simulink model "sampleModel265"  (R2021b)
settings: Solver=VariableStepAuto  StartTime=0.0  StopTime=10.0  RelTol=1e-3
undefined symbols (not defined in the file or in its folder): DiscIntNeverNeededParam, Newton, Raphson
libraries: simulink x9, slpidlib x1
settings Model: Creator=user  LastModifiedBy=user

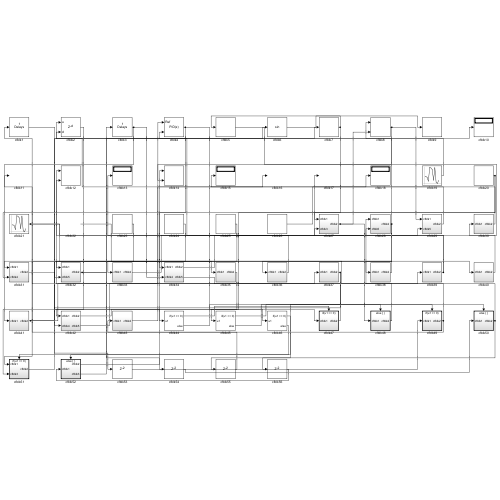
[thumbnail: Simulink's stored preview of the top-level diagram]
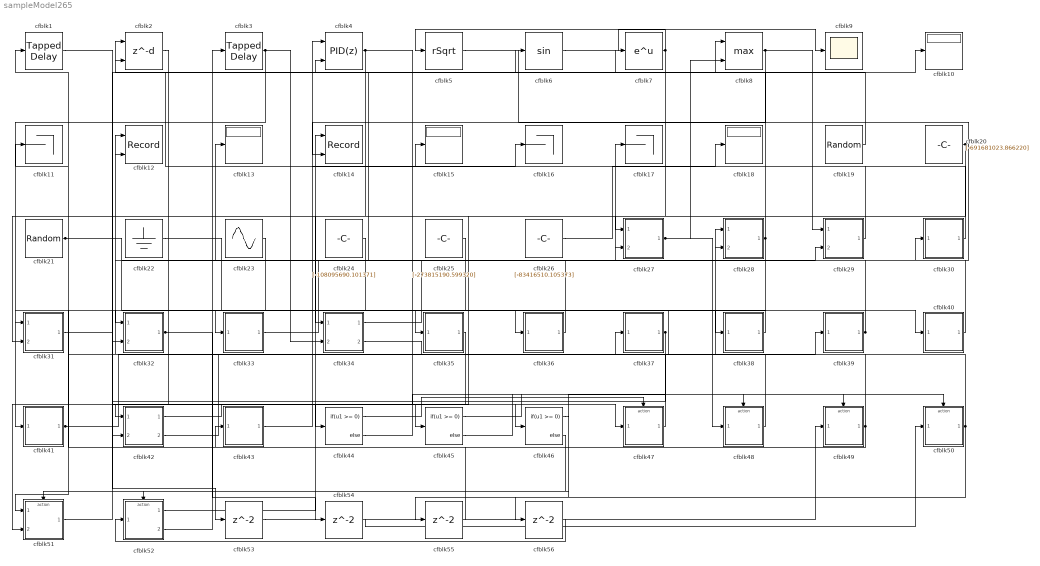
== system sampleModel265 ==
  cfblk1 : simulink/Discrete/Tapped Delay  vinit=0.0  samptime=-1  NumDelays=1  DelayOrder=Oldest  includeCurrent=off
  cfblk{10,13,15,18} (4 alike) : Display
  cfblk11 : Terminator
  cfblk12 : Record  FileSettingsInternal="{\"entries\":[{\"content\":{\"excelSettings\":{\"content\":{},\"type\":\"Streamout.ExcelSettings\"}},\"type\":\"Streamout.FileSettingStorage\",\"uuid\":\"94a5c3c0-ca64-4e36-ac7f-d04636a5f23d\"}],\"packageUris\":[\"http://schema.mathworks.com/mf0/streamout_blocks/R2020a\"],\"version\":\"1.0\"}"  Layout=[1 1]  SignalsInternal="{\"entries\":[{\"content\":{\"signals\":[{\"content\":{\"blockPath\":[\"sampleModel265/cfblk12\"],\"channel\":[],\"dimensions\":[1],\"domain\":\"sampleModel265/cfblk12\",\"lineColor\":\"#a2142f\",\"plots\":[1],\"port\":1,\"sid\":[\"\"],\"signalID\":11021,\"signalName\":\"cfblk47\"},\"type\":\"RecordBlkView.Signal\",\"uuid\":\"85f619e6-c166-47fc-b281-92095b2e0ded\"},{\"content\":{\"blockPath\":[\"sampleModel265/cfblk12\"],\"channel\":[],\"dimensions\":[1],\"domain\":\"sampleModel265/cfblk12\",\"lineColor\":\"#139fff\",\"plots\":[1],\"port\":2,\"sid\":[\"\"],\"signalID\":11025,\"signalName\":\"cfblk40\"},\"type\":\"RecordBlkView.Signal\",\"uuid\":\"cdf1bb3a-11ff-4296-b8df-4a9dbd689937\"}]},\"type\":\"RecordBlkView.InputSignals\",\"uuid\":\"aee0d6e9-f41f-4389-b4de-0f8d12f61657\"}],\"packageUris\":[\"http://schema.mathworks.com/mf0/streamout_blocks/R2020a\"],\"version\":\"1.0\"}"  VisualizationBindings="{\"xyplotplugin\":{\"info\":[{\"series\":[{\"bindingParametersList\":[{\"parameter\":\"X-Axis\",\"signalID\":11021,\"signalName\":\"cfblk47\"},{\"parameter\":\"Y-Axis\",\"signalID\":11025,\"signalName\":\"cfblk40\"}],\"seriesID\":38759}],\"subplotID\":1}]}}"  CompatibilityTag=XY
  cfblk14 : Record  FileSettingsInternal="{\"entries\":[{\"content\":{\"excelSettings\":{\"content\":{},\"type\":\"Streamout.ExcelSettings\"}},\"type\":\"Streamout.FileSettingStorage\",\"uuid\":\"8704c8db-9a0e-4fec-bce2-c10549bc8203\"}],\"packageUris\":[\"http://schema.mathworks.com/mf0/streamout_blocks/R2020a\"],\"version\":\"1.0\"}"  Layout=[1 1]  SignalsInternal="{\"entries\":[{\"content\":{\"signals\":[{\"content\":{\"blockPath\":[\"sampleModel265/cfblk14\"],\"channel\":[],\"dimensions\":[1],\"domain\":\"sampleModel265/cfblk14\",\"lineColor\":\"#a2142f\",\"plots\":[1],\"port\":1,\"sid\":[\"\"],\"signalID\":11029,\"signalName\":\"cfblk52:1\"},\"type\":\"RecordBlkView.Signal\",\"uuid\":\"9f14bc3c-b124-479f-9d7d-5ec5307796c1\"},{\"content\":{\"blockPath\":[\"sampleModel265/cfblk14\"],\"channel\":[],\"dimensions\":[1],\"domain\":\"sampleModel265/cfblk14\",\"lineColor\":\"#139fff\",\"plots\":[1],\"port\":2,\"sid\":[\"\"],\"signalID\":11033,\"signalName\":\"cfblk8\"},\"type\":\"RecordBlkView.Signal\",\"uuid\":\"a3cd0ba9-c32c-4abe-85ac-9eba25fc91aa\"}]},\"type\":\"RecordBlkView.InputSignals\",\"uuid\":\"c0d32c16-2111-47bb-aa87-fac3f9eeb510\"}],\"packageUris\":[\"http://schema.mathworks.com/mf0/streamout_blocks/R2020a\"],\"version\":\"1.0\"}"  VisualizationBindings="{\"xyplotplugin\":{\"info\":[{\"series\":[{\"bindingParametersList\":[{\"parameter\":\"X-Axis\",\"signalID\":11029,\"signalName\":\"cfblk52:1\"},{\"parameter\":\"Y-Axis\",\"signalID\":11033,\"signalName\":\"cfblk8\"}],\"seriesID\":46910}],\"subplotID\":1}]}}"  CompatibilityTag=XY
  cfblk16 : Terminator
  cfblk17 : Terminator
  cfblk19 : RandomNumber  Mean=[-17684.841578]  Variance=[64763.330717]  Seed=[934609408.000000]  SampleTime=0.1
  cfblk2 : Delay  DelayLengthSource=Input port  SampleTime=1
      settings: InputPortMap=u0,p1
  cfblk20 : Constant  Value=[-691681023.866220]  SampleTime=1
  cfblk21 : RandomNumber  Mean=[42362.461850]  Variance=[21600.172597]  Seed=[389411026.000000]  SampleTime=0.1
  cfblk22 : Ground
  cfblk23 : Sin  Amplitude=[904038054.961735]  Bias=[-430535881.463050]  SampleTime=0
  cfblk24 : Constant  Value=[-108095690.101371]  SampleTime=1
  cfblk25 : Constant  Value=[-273815190.599320]  SampleTime=1
  cfblk26 : Constant  Value=[-83416510.105373]  SampleTime=1
  cfblk27 : Subsystem
  cfblk28 : Subsystem
  cfblk29 : Subsystem
  cfblk3 : simulink/Discrete/Tapped Delay  vinit=0.0  samptime=-1  NumDelays=1  DelayOrder=Oldest  includeCurrent=off
  cfblk30 : Subsystem
  cfblk31 : Subsystem
  cfblk32 : Subsystem
  cfblk33 : Subsystem
  cfblk34 : Subsystem
  cfblk35 : Subsystem
  cfblk36 : Subsystem
  cfblk37 : Subsystem
  cfblk38 : Subsystem
  cfblk39 : Subsystem
  cfblk4 : slpidlib/PID Controller (2DOF)  Controller=PID  Form=Parallel  TimeDomain=Discrete-time  UseExternalTs=off  SampleTime=1  IntegratorMethod=Forward Euler  FilterMethod=Forward Euler  ControllerParametersSource=internal  P=1  I=1  D=0  UseFilter=on  N=100  b=1  c=1  TunerSelectOption=Transfer Function Based (PID Tuner App)  InitialConditionSource=internal  InitialConditionForIntegrator=0  InitialConditionForFilter=0  DifferentiatorICPrevScaledInput=0  ExternalReset=none  TrackingMode=off  Kt=1  LimitOutput=off  SatLimitsSource=internal  UpperSaturationLimit=inf  LowerSaturationLimit=-inf  LinearizeAsGain=off  AntiWindupMode=none  Kb=1  POutMin=[]  POutMax=[]  IOutMin=[]  IOutMax=[]  DOutMin=[]  DOutMax=[]  NOutMin=[]  NOutMax=[]  bOutMin=[]  bOutMax=[]  cOutMin=[]  cOutMax=[]  SumOutMin=[]  SumOutMax=[]  SaturationOutMin=[]  SaturationOutMax=[]  PParamMin=[]  PParamMax=[]  IParamMin=[]  IParamMax=[]  DParamMin=[]  DParamMax=[]  NParamMin=[]  NParamMax=[]  bParamMin=[]  bParamMax=[]  cParamMin=[]  cParamMax=[]  KbParamMin=[]  KbParamMax=[]  KtParamMin=[]  KtParamMax=[]  KbOutMin=[]  KbOutMax=[]  KtOutMin=[]  KtOutMax=[]  IntegratorOutMin=[]  IntegratorOutMax=[]  FilterOutMin=[]  FilterOutMax=[]  SumI1OutMin=[]  SumI1OutMax=[]  SumI2OutMin=[]  SumI2OutMax=[]  SumI3OutMin=[]  SumI3OutMax=[]  SumI4OutMin=[]  SumI4OutMax=[]  SumDOutMin=[]  SumDOutMax=[]  Sum1OutMin=[]  Sum1OutMax=[]  Sum2OutMin=[]  Sum2OutMax=[]  Sum3OutMin=[]  Sum3OutMax=[]  DifferentiatorOutMin=[]  DifferentiatorOutMax=[]  FilterDiffOutCoefMin=[]  FilterDiffOutCoefMax=[]  ReciprocalOutMin=[]  ReciprocalOutMax=[]  SumDenOutMin=[]  SumDenOutMax=[]  SumNumOutMin=[]  SumNumOutMax=[]  DivideOutMin=[]  DivideOutMax=[]  UdiffTsProdOutMin=[]  UdiffTsProdOutMax=[]  NTsProdOutMin=[]  NTsProdOutMax=[]  UintegralTsProdOutMin=[]  UintegralTsProdOutMax=[]  UngainTsProdOutMin=[]  UngainTsProdOutMax=[]  IntegratorContinuousStateAttributes=''  IntegratorStateMustResolveToSignalObject=off  IntegratorRTWStateStorageClass=Auto  FilterContinuousStateAttributes=''  FilterStateMustResolveToSignalObject=off  FilterRTWStateStorageClass=Auto  ParallelPVariant=InternalParameters  IdealPVariant=Disabled  IVariant=InternalParameters  DVariant=InternalParameters  bVariant=InternalParameters  cVariant=InternalParameters  IntegratorVariant=Discrete  SatVariant=Disabled  AWVariant=Passthrough  PCopyVariant=Disabled  TRVariant=Disabled  FdbkBlocksVariant=Forward  IdealPFdbkVariant=Disabled  SatFdbkVariant=Disabled  DerivativeFilterVariant=ForwardEulerFilter  NVariant=InternalParameters  NCopyVariant=Disabled  FilterICVariant=InternalICsFilter  IntegratorICVariant=InternalICs  ExternalResetVariant=Disabled  TRSumVariant=Passthrough  SumFdbkVariant=Disabled  SumVariant=Sum_PID  TsampFilterVariant=InternalTs  TsampNgainVariant=Passthrough  TsampIntegralVariant=Passthrough  ExternalSaturationOutDataTypeStr=Inherit: Same as second input
      settings: SourceProductBaseCode=SL
  cfblk40 : Subsystem
  cfblk41 : Subsystem
  cfblk42 : Subsystem
  cfblk43 : Subsystem
  cfblk44 : If  IfExpression=u1 >= 0  SampleTime=1
  cfblk45 : If  IfExpression=u1 >= 0  SampleTime=1
  cfblk46 : If  IfExpression=u1 >= 0  SampleTime=1
  cfblk47 : Subsystem  TreatAsAtomicUnit=on
  cfblk48 : Subsystem  TreatAsAtomicUnit=on
  cfblk49 : Subsystem  TreatAsAtomicUnit=on
  cfblk5 : Sqrt  Operator=rSqrt  AlgorithmType=Newton-Raphson  SaturateOnIntegerOverflow=on
  cfblk50 : Subsystem  TreatAsAtomicUnit=on
  cfblk51 : Subsystem  TreatAsAtomicUnit=on
  cfblk52 : Subsystem  TreatAsAtomicUnit=on
  cfblk{53..56} (4 alike) : Delay  SampleTime=1
  cfblk6 : Trigonometry
  cfblk7 : Math  SaturateOnIntegerOverflow=on
  cfblk8 : MinMax  Function=max  Inputs=2
  cfblk9 : Scope
  wires:
  cfblk47/1(cfblk2) -> cfblk12/1
  cfblk37/1(cfblk2) -> cfblk42/2(cfblk4), cfblk56/1
  cfblk3/1 -> cfblk41/1(cfblk1), cfblk34/2(cfblk4)
  cfblk7/1 -> cfblk5/1, cfblk45/1
  cfblk39/1(cfblk2) -> cfblk17/1, cfblk13/1
  cfblk52/1(cfblk2) -> cfblk14/1
  cfblk34/1(cfblk2) -> cfblk28/1(cfblk1)
  cfblk20/1 -> cfblk27/1(cfblk1), cfblk34/1(cfblk1)
  cfblk42/1(cfblk2) -> cfblk44/1
  cfblk25/1 -> cfblk33/1(cfblk1)
  cfblk5/1 -> cfblk30/1(cfblk1)
  cfblk29/1(cfblk2) -> cfblk2/1
  cfblk49/1(cfblk2) -> cfblk36/1(cfblk1), cfblk43/1(cfblk1)
  cfblk32/1(cfblk2) -> cfblk6/1, cfblk54/1
  cfblk42/2(cfblk5) -> cfblk4/1
  cfblk24/1 -> cfblk31/1(cfblk1)
  cfblk40/1(cfblk2) -> cfblk12/2
  cfblk52/2(cfblk3) -> cfblk3/1
  cfblk30/1(cfblk2) -> cfblk15/1
  cfblk4/1 -> cfblk47/1(cfblk1), cfblk31/2(cfblk4)
  cfblk50/1(cfblk2) -> cfblk28/2(cfblk5), cfblk55/1
  cfblk19/1 -> cfblk2/2
  cfblk6/1 -> cfblk9/1
  cfblk23/1 -> cfblk51/1(cfblk1)
  cfblk34/2(cfblk5) -> cfblk39/1(cfblk1)
  cfblk22/1 -> cfblk35/1(cfblk1)
  cfblk43/1(cfblk2) -> cfblk16/1
  cfblk38/1(cfblk2) -> cfblk32/1(cfblk1)
  cfblk41/1(cfblk2) -> cfblk37/1(cfblk1), cfblk10/1
  cfblk2/1 -> cfblk42/1(cfblk1)
  cfblk8/1 -> cfblk29/1(cfblk1), cfblk14/2
  cfblk35/1(cfblk2) -> cfblk51/2(cfblk3)
  cfblk21/1 -> cfblk40/1(cfblk1), cfblk27/2(cfblk3)
  cfblk33/1(cfblk2) -> cfblk29/2(cfblk5)
  cfblk48/1(cfblk2) -> cfblk11/1
  cfblk36/1(cfblk2) -> cfblk4/2
  cfblk26/1 -> cfblk18/1
  cfblk27/1(cfblk2) -> cfblk48/1(cfblk1), cfblk8/2
  cfblk28/1(cfblk2) -> cfblk32/2(cfblk5), cfblk8/1, cfblk38/1(cfblk1)
  cfblk1/1 -> cfblk46/1
  cfblk51/1(cfblk2) -> cfblk7/1
  cfblk44/1 -> cfblk47/Action
  cfblk44/2 -> cfblk48/Action
  cfblk45/1 -> cfblk49/Action
  cfblk45/2 -> cfblk50/Action
  cfblk46/1 -> cfblk51/Action
  cfblk46/2 -> cfblk52/Action
  cfblk31/1(cfblk2) -> cfblk53/1
  cfblk53/1 -> cfblk49/1(cfblk1)
  cfblk54/1 -> cfblk50/1(cfblk1)
  cfblk55/1 -> cfblk1/1
  cfblk56/1 -> cfblk52/1(cfblk1)

== system sampleModel265/cfblk27 ==
  cfblk1 : Inport
  cfblk3 : Inport  Port=2
  cfblk2 : Outport
  wires:
  cfblk3/1 -> cfblk2/1

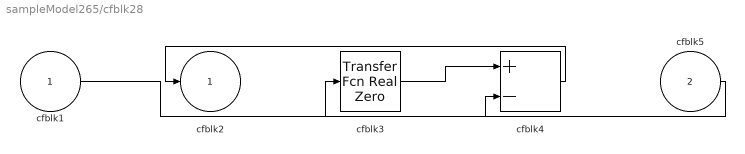
== system sampleModel265/cfblk28 ==
  cfblk1 : Inport
  cfblk5 : Inport  Port=2
  cfblk3 : simulink/Discrete/Transfer Fcn Real Zero  ZeroZ=0.75  ICPrevInput=0.0  DoSatur=off
      settings: SourceProductBaseCode=SL
  cfblk4 : Sum  Inputs=+-
  cfblk2 : Outport
  wires:
  cfblk3/1 -> cfblk4/1
  cfblk4/1 -> cfblk2/1
  cfblk5/1 -> cfblk3/1
  cfblk1/1 -> cfblk4/2

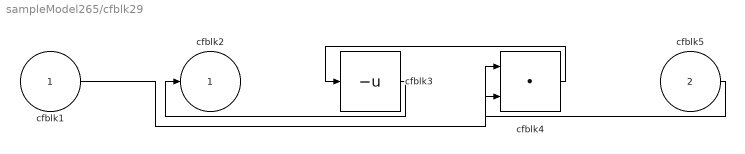
== system sampleModel265/cfblk29 ==
  cfblk1 : Inport
  cfblk5 : Inport  Port=2
  cfblk3 : UnaryMinus
  cfblk4 : DotProduct  InputSameDT=on  OutDataTypeStr=Inherit: Inherit via internal rule
  cfblk2 : Outport
  wires:
  cfblk4/1 -> cfblk3/1
  cfblk3/1 -> cfblk2/1
  cfblk1/1 -> cfblk4/1
  cfblk5/1 -> cfblk4/2

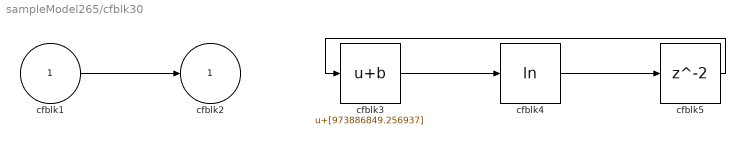
== system sampleModel265/cfblk30 ==
  cfblk1 : Inport
  cfblk3 : Bias  Bias=[973886849.256937]
  cfblk4 : Math  Operator=log  SaturateOnIntegerOverflow=on
  cfblk5 : Delay  SampleTime=1
  cfblk2 : Outport
  wires:
  cfblk3/1 -> cfblk4/1
  cfblk1/1 -> cfblk2/1
  cfblk4/1 -> cfblk5/1
  cfblk5/1 -> cfblk3/1

== system sampleModel265/cfblk31 ==
  cfblk1 : Inport
  cfblk4 : Inport  Port=2
  cfblk3 : Gain  Gain=[624133063.850949]
  cfblk2 : Outport
  wires:
  cfblk1/1 -> cfblk3/1
  cfblk3/1 -> cfblk2/1

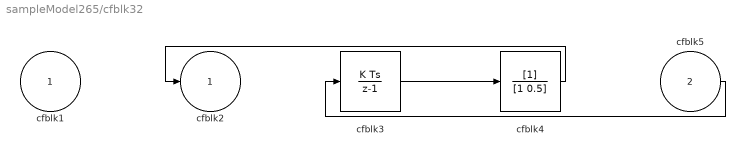
== system sampleModel265/cfblk32 ==
  cfblk1 : Inport
  cfblk5 : Inport  Port=2
  cfblk3 : DiscreteIntegrator  ICPrevOutput=DiscIntNeverNeededParam  ICPrevScaledInput=DiscIntNeverNeededParam
  cfblk4 : DiscreteFilter  SampleTime=1
  cfblk2 : Outport
  wires:
  cfblk4/1 -> cfblk2/1
  cfblk3/1 -> cfblk4/1
  cfblk5/1 -> cfblk3/1

== system sampleModel265/cfblk33 ==
  cfblk1 : Inport
  cfblk3 : simulink/Discrete/Tapped Delay  vinit=0.0  samptime=-1  NumDelays=1  DelayOrder=Oldest  includeCurrent=off
  cfblk4 : Math  Operator=10^u  SaturateOnIntegerOverflow=on
  cfblk2 : Outport
  wires:
  cfblk3/1 -> cfblk2/1
  cfblk4/1 -> cfblk3/1
  cfblk1/1 -> cfblk4/1

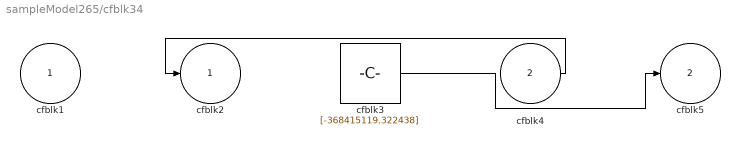
== system sampleModel265/cfblk34 ==
  cfblk1 : Inport
  cfblk4 : Inport  Port=2
  cfblk3 : Constant  Value=[-368415119.322438]  SampleTime=1
  cfblk2 : Outport
  cfblk5 : Outport  Port=2
  wires:
  cfblk4/1 -> cfblk2/1
  cfblk3/1 -> cfblk5/1

== system sampleModel265/cfblk35 ==
  cfblk1 : Inport
  cfblk3 : Abs
  cfblk2 : Outport
  wires:
  cfblk1/1 -> cfblk3/1
  cfblk3/1 -> cfblk2/1

== system sampleModel265/cfblk36 ==
  cfblk1 : Inport
  cfblk3 : Product  Inputs=**
  cfblk2 : Outport
  wires:
  cfblk1/1 -> cfblk3/1, cfblk3/2
  cfblk3/1 -> cfblk2/1

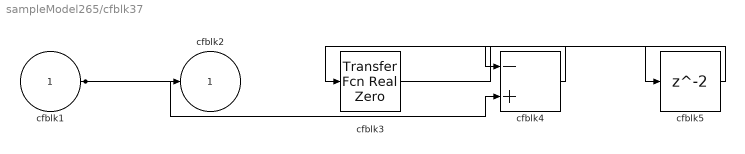
== system sampleModel265/cfblk37 ==
  cfblk1 : Inport
  cfblk3 : simulink/Discrete/Transfer Fcn Real Zero  ZeroZ=0.75  ICPrevInput=0.0  DoSatur=off
      settings: SourceProductBaseCode=SL
  cfblk4 : Sum  Inputs=-+
  cfblk5 : Delay  SampleTime=1
  cfblk2 : Outport
  wires:
  cfblk1/1 -> cfblk4/2, cfblk2/1
  cfblk4/1 -> cfblk3/1
  cfblk3/1 -> cfblk5/1
  cfblk5/1 -> cfblk4/1

== system sampleModel265/cfblk38 ==
  cfblk1 : Inport
  cfblk3 : Product  Inputs=*
  cfblk2 : Outport
  wires:
  cfblk1/1 -> cfblk3/1
  cfblk3/1 -> cfblk2/1

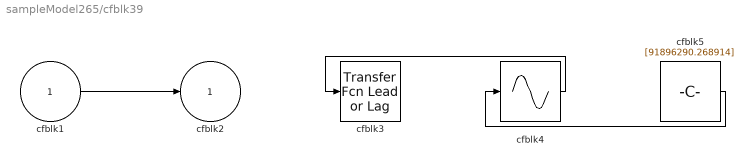
== system sampleModel265/cfblk39 ==
  cfblk1 : Inport
  cfblk3 : simulink/Discrete/Transfer Fcn Lead or Lag  PoleZ=0.95  ZeroZ=0.75  ICPrevOutput=0.0  ICPrevInput=0.0  DoSatur=off
      settings: SourceProductBaseCode=SL
  cfblk4 : Sin  TimeSource=Use external signal  SampleTime=0
  cfblk5 : Constant  Value=[91896290.268914]  SampleTime=1
  cfblk2 : Outport
  wires:
  cfblk1/1 -> cfblk2/1
  cfblk4/1 -> cfblk3/1
  cfblk5/1 -> cfblk4/1

== system sampleModel265/cfblk40 ==
  cfblk1 : Inport
  cfblk3 : simulink/Math Operations/MinMax Running Resettable  Function=min  vinit=0.0
  cfblk2 : Outport
  wires:
  cfblk1/1 -> cfblk3/1, cfblk3/2
  cfblk3/1 -> cfblk2/1

== system sampleModel265/cfblk41 ==
  cfblk1 : Inport
  cfblk3 : simulink/Discrete/Tapped Delay  vinit=0.0  samptime=-1  NumDelays=1  DelayOrder=Oldest  includeCurrent=off
  cfblk4 : UnaryMinus
  cfblk2 : Outport
  wires:
  cfblk1/1 -> cfblk3/1
  cfblk3/1 -> cfblk4/1
  cfblk4/1 -> cfblk2/1

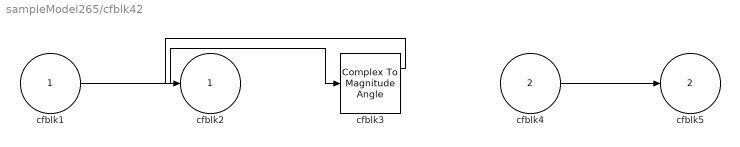
== system sampleModel265/cfblk42 ==
  cfblk1 : Inport
  cfblk4 : Inport  Port=2
  cfblk3 : ComplexToMagnitudeAngle
  cfblk2 : Outport
  cfblk5 : Outport  Port=2
  wires:
  cfblk1/1 -> cfblk3/1
  cfblk3/1 -> cfblk2/1
  cfblk4/1 -> cfblk5/1

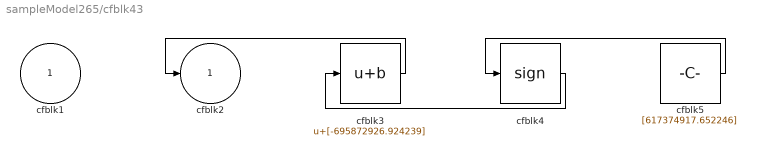
== system sampleModel265/cfblk43 ==
  cfblk1 : Inport
  cfblk3 : Bias  Bias=[-695872926.924239]
  cfblk4 : Signum
  cfblk5 : Constant  Value=[617374917.652246]  SampleTime=1
  cfblk2 : Outport
  wires:
  cfblk3/1 -> cfblk2/1
  cfblk4/1 -> cfblk3/1
  cfblk5/1 -> cfblk4/1

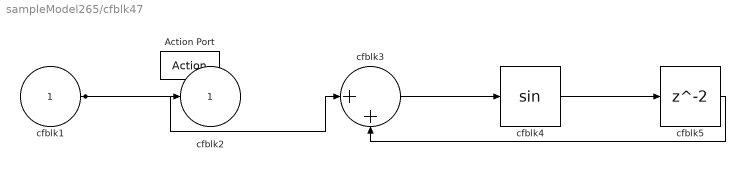
== system sampleModel265/cfblk47 ==
  cfblk1 : Inport
  Action Port : ActionPort  ActionPortLabel=if(u1 >= 0)
  cfblk3 : Sum  Inputs=|++
  cfblk4 : Trigonometry
  cfblk5 : Delay
  cfblk2 : Outport
  wires:
  cfblk3/1 -> cfblk4/1
  cfblk1/1 -> cfblk3/1, cfblk2/1
  cfblk4/1 -> cfblk5/1
  cfblk5/1 -> cfblk3/2

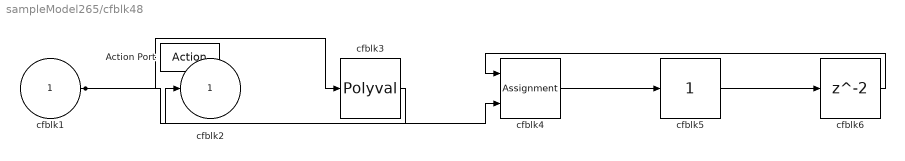
== system sampleModel265/cfblk48 ==
  cfblk1 : Inport
  Action Port : ActionPort  ActionPortLabel=else
  cfblk3 : Polyval  Coefs=[ +2.081618890e-019, -1.441693666e-014, +4.719686976e-010, -8.536869453e-006, +1.621573104e-001, -8.087801117e+001 ]
  cfblk4 : Assignment  DiagnosticForDimensions=Warning  IndexOptions=Index vector (dialog)  Indices=1  OutputSizes=1
  cfblk5 : simulink/Math Operations/Slider Gain  gain=1  low=0  high=2
  cfblk6 : Delay
  cfblk2 : Outport
  wires:
  cfblk3/1 -> cfblk2/1
  cfblk1/1 -> cfblk3/1, cfblk4/2
  cfblk4/1 -> cfblk5/1
  cfblk5/1 -> cfblk6/1
  cfblk6/1 -> cfblk4/1

== system sampleModel265/cfblk49 ==
  cfblk1 : Inport
  Action Port : ActionPort  ActionPortLabel=if(u1 >= 0)
  cfblk3 : MinMax
  cfblk2 : Outport
  wires:
  cfblk3/1 -> cfblk2/1
  cfblk1/1 -> cfblk3/1

== system sampleModel265/cfblk50 ==
  cfblk1 : Inport
  Action Port : ActionPort  ActionPortLabel=else
  cfblk3 : Constant  Value=[855989115.149519]  SampleTime=1
  cfblk2 : Outport
  wires:
  cfblk3/1 -> cfblk2/1

== system sampleModel265/cfblk51 ==
  cfblk1 : Inport
  cfblk3 : Inport  Port=2
  Action Port : ActionPort  ActionPortLabel=if(u1 >= 0)
  cfblk2 : Outport
  wires:
  cfblk1/1 -> cfblk2/1

== system sampleModel265/cfblk52 ==
  cfblk1 : Inport
  Action Port : ActionPort  ActionPortLabel=else
  cfblk2 : Outport
  cfblk3 : Outport  Port=2
  wires:
  cfblk1/1 -> cfblk3/1, cfblk2/1
